simulink model "turbfbDs"  (R2018a)
settings: Solver=VariableStepAuto  StartTime=0.0  StopTime=10.0  RelTol=1e-3
libraries: simulink x1
settings Model: Creator=mengc  LastModifiedBy=Ducted Fan

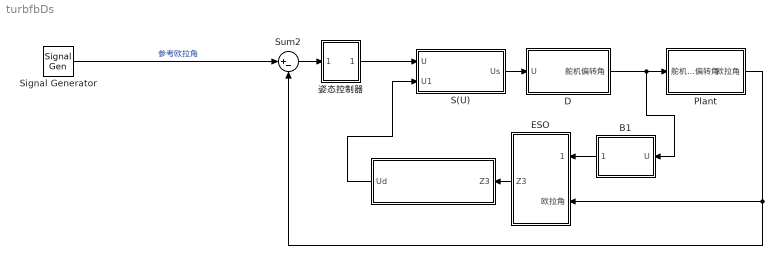
== system turbfbDs ==
  " " : Subsystem
      mask Display:
      | disp('U_d=I(K_0D_s)^+z_3','texmode','on')
      | port_label('input',1,'\it{z_3}','texmode','on');
      | port_label('output',1,'\it{U_d}','texmode','on');
  B1 : Subsystem
      mask Display:
      | port_label('input',1,'\it{\delta}','texmode','on');
      | port_label('output',1,'\it{I^{-1}K_0\delta}','texmode','on');
  D : Subsystem
      mask Display:
      | disp('\delta=D_sU_s','texmode','on')
      | port_label('input',1,'\it{U_s}','texmode','on');
      | port_label('output',1,'\it{\delta}','texmode','on');
  ESO : Subsystem
      mask Display:
      | port_label('output',1,'\it{z_3}','texmode','on');
      | port_label('input',1,'\it{I^{-1}K_0\delta}','texmode','on');
      | port_label('input',2,'\it{[\phi \theta \psi]^T}','texmode','on');
  Plant : Subsystem
      mask Display:
      | port_label('input',1,'\it{\delta}','texmode','on');
      | port_label('output',1,'\it{[\phi \theta \psi]^T}','texmode','on');
  S(U) : Subsystem
      mask Display:
      | disp('U_s=S(U)','texmode','on')
      | port_label('input',1,'\it{U}','texmode','on');
      | port_label('input',2,'\it{U_d}','texmode','on');
      | port_label('output',1,'\it{U_s}','texmode','on');
  Signal Generator : SignalGenerator  Units=rad/sec
  Sum2 : Sum  Inputs=|+-
  姿态控制器 : Subsystem
      mask Display:
      | port_label('input',1,'\it{e}','texmode','on');
      | port_label('output',1,'\it{U_0}','texmode','on');
  wires:
  ESO/1(Z3) -> " "/1(Z3)
  Plant/1(欧拉角) -> Sum2/2, ESO/2(欧拉角)
  D/1(舵机偏转角) -> Plant/1("舵机偏转角 "), B1/1("U ")
  Sum2/1 -> 姿态控制器/1(误差)
  姿态控制器/1(Uo) -> S(U)/1(U)
  S(U)/1(Us) -> D/1(U)
  B1/1(" ") -> ESO/1(" ")
  " "/1(Ud) -> S(U)/2(U1)
  Signal Generator/1 -> Sum2/1  "参考欧拉角"

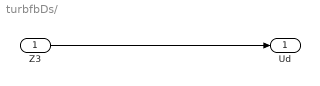
== system turbfbDs/  ==
  Z3 : Inport
  Ud : Outport
  wires:
  Z3/1 -> Ud/1

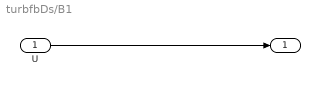
== system turbfbDs/B1 ==
  "U " : Inport
  " " : Outport
  wires:
  "U "/1 -> " "/1

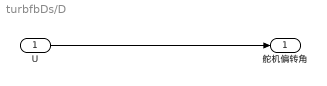
== system turbfbDs/D ==
  U : Inport
  舵机偏转角 : Outport
  wires:
  U/1 -> 舵机偏转角/1

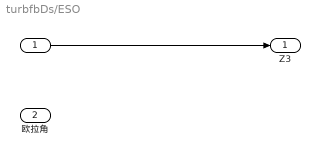
== system turbfbDs/ESO ==
  " " : Inport
  欧拉角 : Inport  Port=2
  Z3 : Outport
  wires:
  " "/1 -> Z3/1

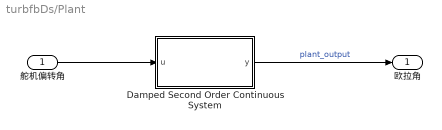
== system turbfbDs/Plant ==
  "舵机偏转角 " : Inport
  Damped Second Order Continuous System : Subsystem  mask{wn=16, zeta=0.6}
      mask prompts: wn "Undamped natural frequency (wn, rad/s)"; zeta "Damping factor (zeta)"
  欧拉角 : Outport
  wires:
  "舵机偏转角 "/1 -> Damped Second Order Continuous System/1(u)
  Damped Second Order Continuous System/1(y) -> 欧拉角/1  "plant_output"

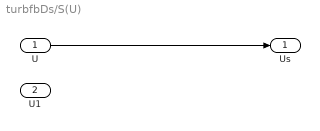
== system turbfbDs/S(U) ==
  U : Inport
  U1 : Inport  Port=2
  Us : Outport
  wires:
  U/1 -> Us/1

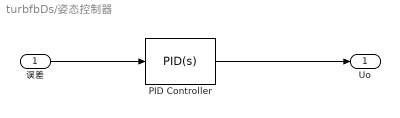
== system turbfbDs/姿态控制器 ==
  误差 : Inport
  PID Controller : simulink/Continuous/PID Controller  Controller=PID  TimeDomain=Continuous-time  SampleTime=-1  IntegratorMethod=Forward Euler  FilterMethod=Forward Euler  Form=Parallel  UseFilter=on  ControllerParametersSource=internal  P=1.2  I=22  D=0.02  N=20  InitialConditionSource=internal  InitialConditionForIntegrator=0  InitialConditionForFilter=0  ExternalReset=none  LimitOutput=off  UpperSaturationLimit=inf  LowerSaturationLimit=-inf  LinearizeAsGain=on  AntiWindupMode=none  Kb=1  TrackingMode=off  Kt=1  PParamMin=[]  PParamMax=[]  IParamMin=[]  IParamMax=[]  DParamMin=[]  DParamMax=[]  NParamMin=[]  NParamMax=[]  KbParamMin=[]  KbParamMax=[]  KtParamMin=[]  KtParamMax=[]  POutMin=[]  POutMax=[]  IOutMin=[]  IOutMax=[]  DOutMin=[]  DOutMax=[]  NOutMin=[]  NOutMax=[]  KbOutMin=[]  KbOutMax=[]  KtOutMin=[]  KtOutMax=[]  IntegratorOutMin=[]  IntegratorOutMax=[]  FilterOutMin=[]  FilterOutMax=[]  SumOutMin=[]  SumOutMax=[]  SumI1OutMin=[]  SumI1OutMax=[]  SumI2OutMin=[]  SumI2OutMax=[]  SumI3OutMin=[]  SumI3OutMax=[]  SumDOutMin=[]  SumDOutMax=[]  SaturationOutMin=[]  SaturationOutMax=[]  IntegratorContinuousStateAttributes=''  IntegratorStateMustResolveToSignalObject=off  IntegratorRTWStateStorageClass=Auto  FilterContinuousStateAttributes=''  FilterStateMustResolveToSignalObject=off  FilterRTWStateStorageClass=Auto  DifferentiatorICPrevScaledInput=0  DifferentiatorOutMin=[]  DifferentiatorOutMax=[]  FilterDiffOutCoefMin=[]  FilterDiffOutCoefMax=[]  SumDenOutMin=[]  SumDenOutMax=[]  SumNumOutMin=[]  SumNumOutMax=[]  ReciprocalOutMin=[]  ReciprocalOutMax=[]  DivideOutMin=[]  DivideOutMax=[]  TunerSelectOption=Transfer Function Based (PID Tuner App)
  Uo : Outport
  wires:
  误差/1 -> PID Controller/1
  PID Controller/1 -> Uo/1

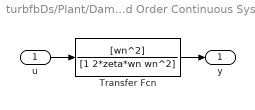
== system turbfbDs/Plant/Damped Second Order Continuous System ==
  u : Inport
  Transfer Fcn : TransferFcn  Numerator=[wn^2]  Denominator=[1 2*zeta*wn wn^2]
  y : Outport
  wires:
  Transfer Fcn/1 -> y/1
  u/1 -> Transfer Fcn/1
